simulink model "testmdl1_mdl"  (Simulink 8.8)
settings: Solver=VariableStepAuto  StartTime=0.0  StopTime=10.0  RelTol=1e-3
settings Model: Creator=sgopalswamy  LastModifiedBy=sgopalswamy
settings DataIOCC: SaveFormat=Dataset  SignalLoggingSaveFormat=Dataset  SaveOutput=off  SaveTime=off
settings OptimizationCC: BlockReduction=off  BooleanDataType=off
settings DebuggingCC: SaveWithParameterizedLinksMsg=none  SignalResolutionControl=TryResolveAllWithWarning  FcnCallInpInsideContextMsg=error  AllowSymbolicDim=off  StateNameClashWarn=none
settings HardwareCC: ProdBitPerPointer=64  ProdBitPerSizeT=64  ProdBitPerPtrDiffT=64  ProdLargestAtomicFloat=Float  ProdIntDivRoundTo=Zero  ProdEndianess=LittleEndian  ProdWordSize=64  ProdHWDeviceType=Intel->x86-64 (Windows64)  TargetUnknown=on
settings ModelReferenceCC: PropagateSignalLabelsOutOfModel=on
settings GRTTargetCC: CombineOutputUpdateFcns=on  GRTInterface=off
settings ConfigComp: CovMetricSettings=dwe  CovHtmlReporting=off  CovSaveCumulativeToWorkspaceVar=off  CovSaveSingleToWorkspaceVar=off  CovExternalEMLEnable=on

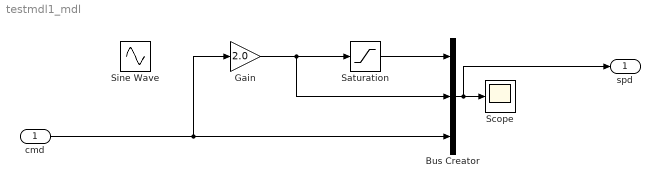
== system testmdl1_mdl ==
  cmd : Inport
  Bus Creator : BusCreator  Inputs=3
  Gain : Gain  Gain=2.0
  Saturation : Saturate
  Scope : Scope
  Sine Wave : Sin  SampleTime=0
  spd : Outport
  wires:
  Gain/1 -> Bus Creator/2, Saturation/1
  Bus Creator/1 -> spd/1, Scope/1
  Saturation/1 -> Bus Creator/1
  cmd/1 -> Bus Creator/3, Gain/1
